simulink library "jcw"  (Simulink 8.1)
settings: Solver=ode45  StartTime=0.0  StopTime=10.0  RelTol=1e-3
libraries: ftc x1, fac x1, fdc x1, fen x1, foc x1, fsr x1
settings Model: Creator=xsellart  LastModifiedBy=xsellart

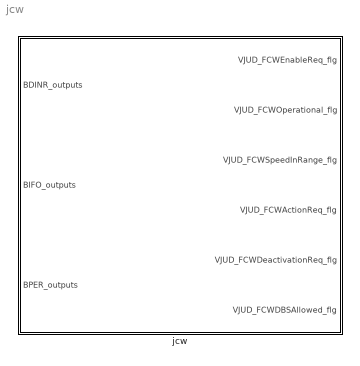
== system jcw ==
  jcw : Subsystem

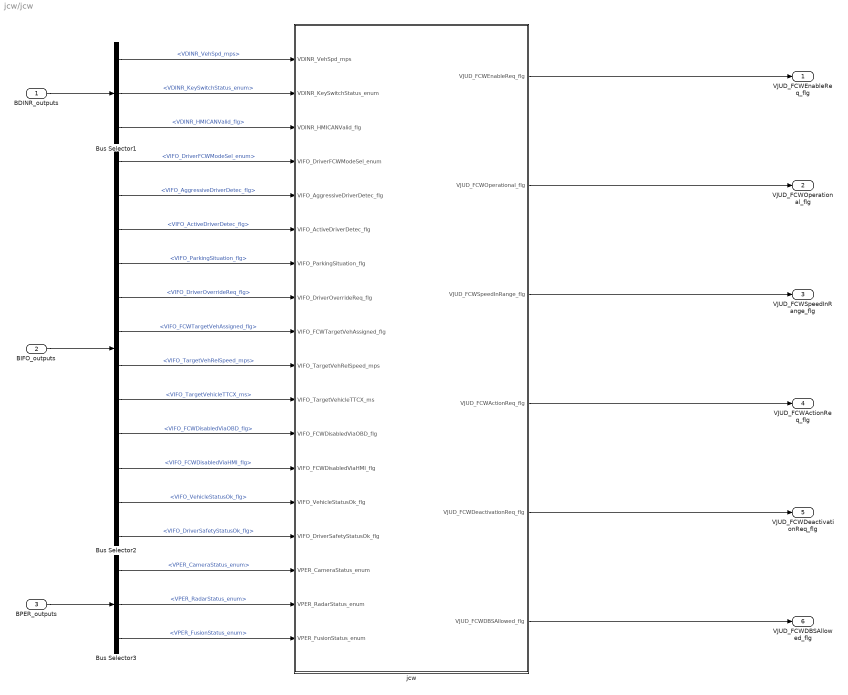
== system jcw/jcw ==
  BDINR_outputs : Inport  OutDataTypeStr=Bus: BDINR_outputs
  BIFO_outputs : Inport  Port=2  OutDataTypeStr=Bus: BIFO_outputs
  BPER_outputs : Inport  Port=3  OutDataTypeStr=Bus: BPER_outputs
  Bus Selector1 : BusSelector  OutputSignals=VDINR_VehSpd_mps,VDINR_KeySwitchStatus_enum,VDINR_HMICANValid_flg
  Bus Selector2 : BusSelector  OutputSignals=VIFO_DriverFCWModeSel_enum,VIFO_AggressiveDriverDetec_flg,VIFO_ActiveDriverDetec_flg,VIFO_ParkingSituation_flg,VIFO_DriverOverrideReq_flg,VIFO_FCWTargetVehAssigned_flg,VIFO_TargetVehRelSpeed_mps,VIFO_TargetVehicleTTCX_ms,VIFO_FCWDisabledViaOBD_flg,VIFO_FCWDisabledViaHMI_flg,VIFO_VehicleStatusOk_flg,VIFO_DriverSafetyStatusOk_flg
  Bus Selector3 : BusSelector  OutputSignals=VPER_CameraStatus_enum,VPER_RadarStatus_enum,VPER_FusionStatus_enum
  jcw : Subsystem
  VJUD_FCWEnableReq_flg : Outport
  VJUD_FCWOperational_flg : Outport  Port=2
  VJUD_FCWSpeedInRange_flg : Outport  Port=3
  VJUD_FCWActionReq_flg : Outport  Port=4
  VJUD_FCWDeactivationReq_flg : Outport  Port=5
  VJUD_FCWDBSAllowed_flg : Outport  Port=6
  wires:
  jcw/3(VJUD_FCWSpeedInRange_flg) -> VJUD_FCWSpeedInRange_flg/1
  jcw/5(VJUD_FCWDeactivationReq_flg) -> VJUD_FCWDeactivationReq_flg/1
  jcw/2(VJUD_FCWOperational_flg) -> VJUD_FCWOperational_flg/1
  jcw/4(VJUD_FCWActionReq_flg) -> VJUD_FCWActionReq_flg/1
  jcw/6(VJUD_FCWDBSAllowed_flg) -> VJUD_FCWDBSAllowed_flg/1
  jcw/1(VJUD_FCWEnableReq_flg) -> VJUD_FCWEnableReq_flg/1
  Bus Selector2/10 -> jcw/13(VIFO_FCWDisabledViaHMI_flg)  "<VIFO_FCWDisabledViaHMI_flg>"
  BPER_outputs/1 -> Bus Selector3/1
  Bus Selector2/11 -> jcw/14(VIFO_VehicleStatusOk_flg)  "<VIFO_VehicleStatusOk_flg>"
  Bus Selector2/9 -> jcw/12(VIFO_FCWDisabledViaOBD_flg)  "<VIFO_FCWDisabledViaOBD_flg>"
  Bus Selector2/12 -> jcw/15(VIFO_DriverSafetyStatusOk_flg)  "<VIFO_DriverSafetyStatusOk_flg>"
  BDINR_outputs/1 -> Bus Selector1/1
  BIFO_outputs/1 -> Bus Selector2/1
  Bus Selector2/6 -> jcw/9(VIFO_FCWTargetVehAssigned_flg)  "<VIFO_FCWTargetVehAssigned_flg>"
  Bus Selector2/7 -> jcw/10(VIFO_TargetVehRelSpeed_mps)  "<VIFO_TargetVehRelSpeed_mps>"
  Bus Selector2/3 -> jcw/6(VIFO_ActiveDriverDetec_flg)  "<VIFO_ActiveDriverDetec_flg>"
  Bus Selector2/4 -> jcw/7(VIFO_ParkingSituation_flg)  "<VIFO_ParkingSituation_flg>"
  Bus Selector2/1 -> jcw/4(VIFO_DriverFCWModeSel_enum)  "<VIFO_DriverFCWModeSel_enum>"
  Bus Selector2/2 -> jcw/5(VIFO_AggressiveDriverDetec_flg)  "<VIFO_AggressiveDriverDetec_flg>"
  Bus Selector2/5 -> jcw/8(VIFO_DriverOverrideReq_flg)  "<VIFO_DriverOverrideReq_flg>"
  Bus Selector2/8 -> jcw/11(VIFO_TargetVehicleTTCX_ms)  "<VIFO_TargetVehicleTTCX_ms>"
  Bus Selector3/2 -> jcw/17(VPER_RadarStatus_enum)  "<VPER_RadarStatus_enum>"
  Bus Selector1/2 -> jcw/2(VDINR_KeySwitchStatus_enum)  "<VDINR_KeySwitchStatus_enum>"
  Bus Selector3/1 -> jcw/16(VPER_CameraStatus_enum)  "<VPER_CameraStatus_enum>"
  Bus Selector1/3 -> jcw/3(VDINR_HMICANValid_flg)  "<VDINR_HMICANValid_flg>"
  Bus Selector3/3 -> jcw/18(VPER_FusionStatus_enum)  "<VPER_FusionStatus_enum>"
  Bus Selector1/1 -> jcw/1(VDINR_VehSpd_mps)  "<VDINR_VehSpd_mps>"

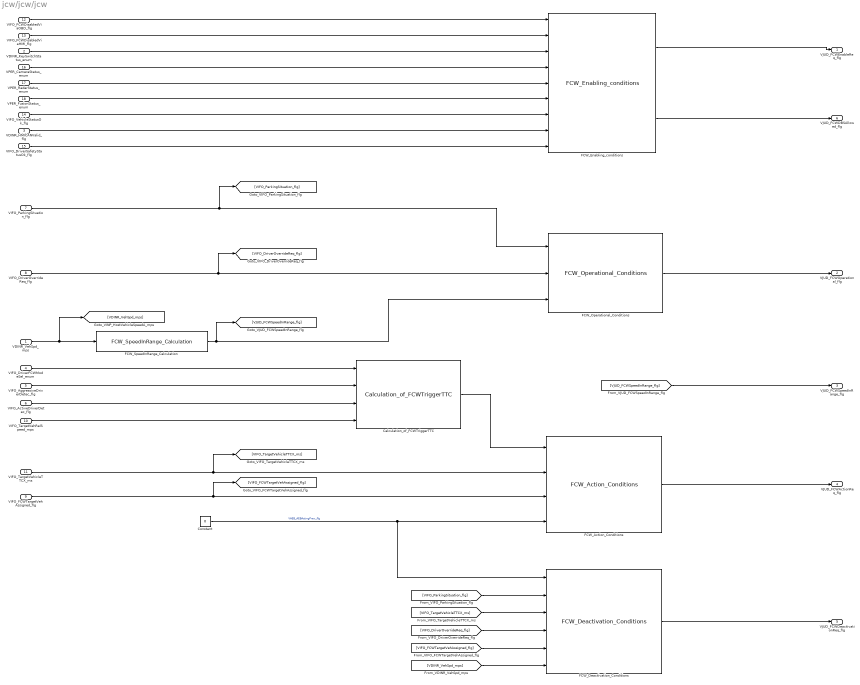
== system jcw/jcw/jcw ==
  VDINR_VehSpd_mps : Inport
  VDINR_KeySwitchStatus_enum : Inport  Port=2
  VDINR_HMICANValid_flg : Inport  Port=3
  VIFO_DriverFCWModeSel_enum : Inport  Port=4
  VIFO_AggressiveDriverDetec_flg : Inport  Port=5
  VIFO_ActiveDriverDetec_flg : Inport  Port=6
  VIFO_ParkingSituation_flg : Inport  Port=7
  VIFO_DriverOverrideReq_flg : Inport  Port=8
  VIFO_FCWTargetVehAssigned_flg : Inport  Port=9
  VIFO_TargetVehRelSpeed_mps : Inport  Port=10
  VIFO_TargetVehicleTTCX_ms : Inport  Port=11
  VIFO_FCWDisabledViaOBD_flg : Inport  Port=12
  VIFO_FCWDisabledViaHMI_flg : Inport  Port=13
  VIFO_VehicleStatusOk_flg : Inport  Port=14
  VIFO_DriverSafetyStatusOk_flg : Inport  Port=15
  VPER_CameraStatus_enum : Inport  Port=16
  VPER_RadarStatus_enum : Inport  Port=17
  VPER_FusionStatus_enum : Inport  Port=18
  Calculation_of_FCWTriggerTTC : ftc/Calculation_of_FCWTriggerTTC
  Constant : Constant  Value=0
  FCW_Action_Conditions : fac/FCW_Action_Conditions
  FCW_Deactivation_Conditions : fdc/FCW_Deactivation_Conditions
  FCW_Enabling_conditions : fen/FCW_Enabling_conditions
  FCW_Operational_Conditions : foc/FCW_Operational_Conditions
  FCW_SpeedInRange_Calculation : fsr/FCW_SpeedInRange_Calculation
  VJUD_FCWEnableReq_flg : Outport
  VJUD_FCWOperational_flg : Outport  Port=2
  VJUD_FCWSpeedInRange_flg : Outport  Port=3
  VJUD_FCWActionReq_flg : Outport  Port=4
  VJUD_FCWDeactivationReq_flg : Outport  Port=5
  VJUD_FCWDBSAllowed_flg : Outport  Port=6
  wires:
  VIFO_TargetVehRelSpeed_mps/1 -> Calculation_of_FCWTriggerTTC/4
  VIFO_ParkingSituation_flg/1 -> FCW_Operational_Conditions/1, [VIFO_ParkingSituation_flg]
  VIFO_DriverOverrideReq_flg/1 -> FCW_Operational_Conditions/2, [VIFO_DriverOverrideReq_flg]
  FCW_SpeedInRange_Calculation/1 -> FCW_Operational_Conditions/3, [VJUD_FCWSpeedInRange_flg]
  VDINR_VehSpd_mps/1 -> FCW_SpeedInRange_Calculation/1, [VDINR_VehSpd_mps]
  [VDINR_VehSpd_mps] -> FCW_Deactivation_Conditions/6
  FCW_Enabling_conditions/2 -> VJUD_FCWDBSAllowed_flg/1
  VPER_RadarStatus_enum/1 -> FCW_Enabling_conditions/5
  VPER_FusionStatus_enum/1 -> FCW_Enabling_conditions/6
  VDINR_HMICANValid_flg/1 -> FCW_Enabling_conditions/8
  VIFO_VehicleStatusOk_flg/1 -> FCW_Enabling_conditions/7
  VPER_CameraStatus_enum/1 -> FCW_Enabling_conditions/4
  VIFO_DriverSafetyStatusOk_flg/1 -> FCW_Enabling_conditions/9
  VDINR_KeySwitchStatus_enum/1 -> FCW_Enabling_conditions/3
  VIFO_FCWDisabledViaHMI_flg/1 -> FCW_Enabling_conditions/2
  VIFO_FCWDisabledViaOBD_flg/1 -> FCW_Enabling_conditions/1
  [VIFO_FCWTargetVehAssigned_flg] -> FCW_Deactivation_Conditions/5
  Constant/1 -> FCW_Action_Conditions/4, FCW_Deactivation_Conditions/1  "VAEB_AEBActingPrev_flg"
  [VJUD_FCWSpeedInRange_flg] -> VJUD_FCWSpeedInRange_flg/1
  FCW_Deactivation_Conditions/1 -> VJUD_FCWDeactivationReq_flg/1
  [VIFO_DriverOverrideReq_flg] -> FCW_Deactivation_Conditions/4
  [VIFO_TargetVehicleTTCX_ms] -> FCW_Deactivation_Conditions/3
  [VIFO_ParkingSituation_flg] -> FCW_Deactivation_Conditions/2
  FCW_Action_Conditions/1 -> VJUD_FCWActionReq_flg/1
  FCW_Operational_Conditions/1 -> VJUD_FCWOperational_flg/1
  Calculation_of_FCWTriggerTTC/1 -> FCW_Action_Conditions/1
  VIFO_ActiveDriverDetec_flg/1 -> Calculation_of_FCWTriggerTTC/3
  VIFO_AggressiveDriverDetec_flg/1 -> Calculation_of_FCWTriggerTTC/2
  VIFO_DriverFCWModeSel_enum/1 -> Calculation_of_FCWTriggerTTC/1
  VIFO_TargetVehicleTTCX_ms/1 -> [VIFO_TargetVehicleTTCX_ms], FCW_Action_Conditions/2
  VIFO_FCWTargetVehAssigned_flg/1 -> [VIFO_FCWTargetVehAssigned_flg], FCW_Action_Conditions/3
  FCW_Enabling_conditions/1 -> VJUD_FCWEnableReq_flg/1
